simulink library "pid_controller_lib"  (R2025b)
settings: Solver=VariableStepAuto  StartTime=0.0  StopTime=10.0  RelTol=1e-3
settings Model: Creator=ali89  LastModifiedBy=ali89

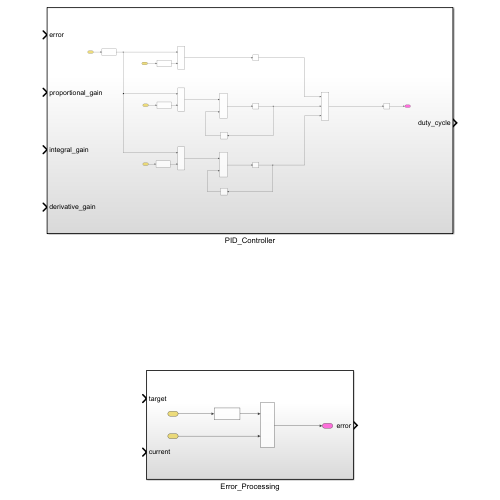
[thumbnail: Simulink's stored preview of the top-level diagram]
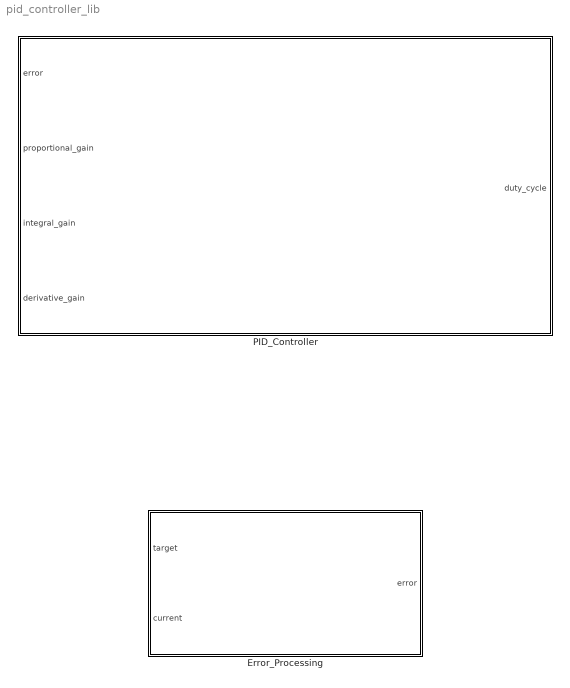
== system pid_controller_lib ==
  Error_Processing : Subsystem
  PID_Controller : Subsystem

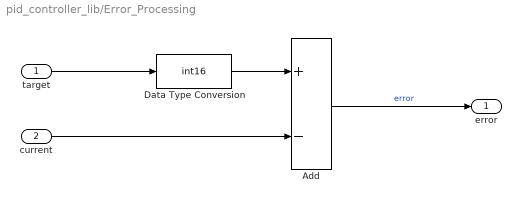
== system pid_controller_lib/Error_Processing ==
  target : Inport
  current : Inport  Port=2
  Add : Sum  Inputs=+-
  Data Type Conversion : DataTypeConversion  OutDataTypeStr=int16  SaturateOnIntegerOverflow=off  RndMeth=Floor
  error : Outport
  wires:
  current/1 -> Add/2
  target/1 -> Data Type Conversion/1
  Add/1 -> error/1  "error"
  Data Type Conversion/1 -> Add/1

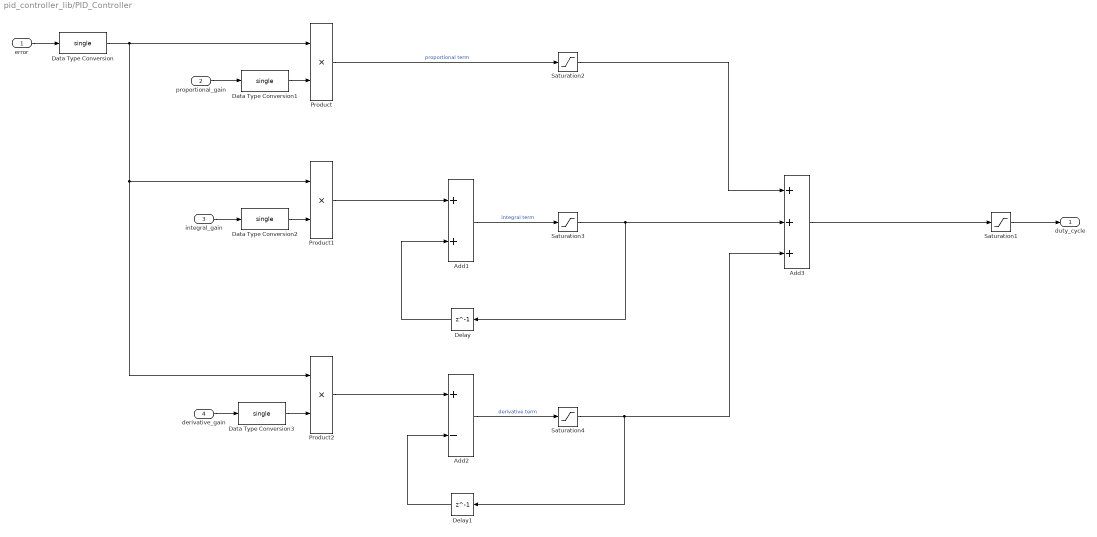
== system pid_controller_lib/PID_Controller ==
  error : Inport
  proportional_gain : Inport  Port=2
  integral_gain : Inport  Port=3
  derivative_gain : Inport  Port=4
  Add1 : Sum
  Add2 : Sum  Inputs=+-
  Add3 : Sum  Inputs=+++
  Data Type Conversion{,1..3} (4 alike) : DataTypeConversion  OutDataTypeStr=single  SaturateOnIntegerOverflow=off  RndMeth=Floor
  Delay : Delay  DelayLength=1  InputProcessing=Columns as channels (frame based)
  Delay1 : Delay  DelayLength=1  InputProcessing=Columns as channels (frame based)
  Product : Product
  Product1 : Product
  Product2 : Product
  Saturation1 : Saturate  UpperLimit=255  LowerLimit=0
  Saturation2 : Saturate  UpperLimit=255  LowerLimit=-255
  Saturation3 : Saturate  UpperLimit=255  LowerLimit=-255
  Saturation4 : Saturate  UpperLimit=255  LowerLimit=-255
  duty_cycle : Outport
  wires:
  Data Type Conversion3/1 -> Product2/2
  Data Type Conversion2/1 -> Product1/2
  Data Type Conversion1/1 -> Product/2
  Data Type Conversion/1 -> Product/1, Product1/1, Product2/1
  Saturation4/1 -> Add3/3, Delay1/1
  Add2/1 -> Saturation4/1  "derivative term"
  derivative_gain/1 -> Data Type Conversion3/1
  Add1/1 -> Saturation3/1  "integral term"
  Delay/1 -> Add1/2
  Product2/1 -> Add2/1
  error/1 -> Data Type Conversion/1
  integral_gain/1 -> Data Type Conversion2/1
  Saturation3/1 -> Add3/2, Delay/1
  Product1/1 -> Add1/1
  proportional_gain/1 -> Data Type Conversion1/1
  Saturation1/1 -> duty_cycle/1
  Delay1/1 -> Add2/2
  Saturation2/1 -> Add3/1
  Product/1 -> Saturation2/1  "proportional term"
  Add3/1 -> Saturation1/1
